simulink model "cntctr"  (R2023b)
settings: Solver=FixedStepDiscrete  StartTime=0.0  StopTime=10.0  FixedStep=0.01  RelTol=1e-3
settings Model: Creator=OWNER  LastModifiedBy=OWNER

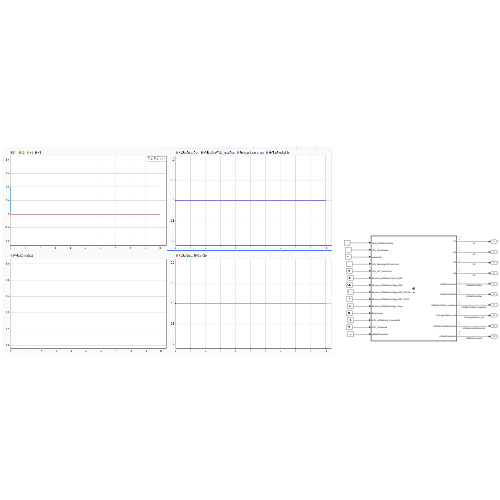
[thumbnail: Simulink's stored preview of the top-level diagram]
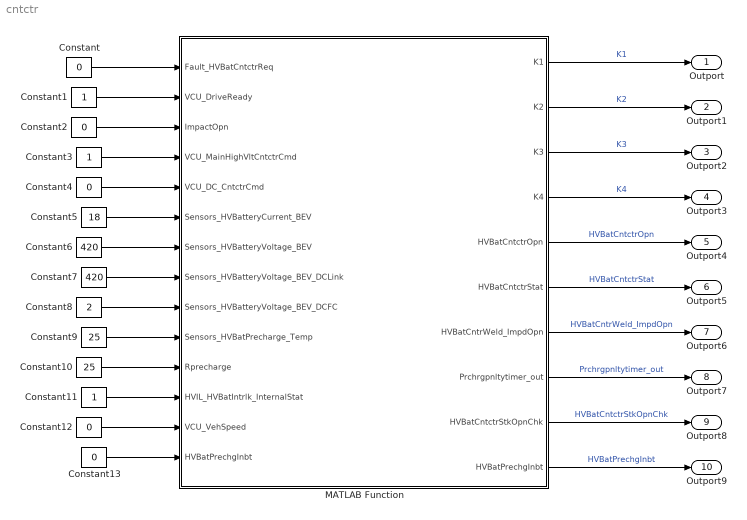
== system cntctr ==
  Constant{,2,4,12..13} (5 alike) : Constant  Value=0
  Constant1 : Constant
  Constant10 : Constant  Value=25
  Constant11 : Constant
  Constant3 : Constant
  Constant5 : Constant  Value=18
  Constant6 : Constant  Value=420
  Constant7 : Constant  Value=420
  Constant8 : Constant  Value=2
  Constant9 : Constant  Value=25
  MATLAB Function : MATLAB Function  TreatAsAtomicUnit=on
  Outport : Outport
  Outport1 : Outport  Port=2
  Outport2 : Outport  Port=3
  Outport3 : Outport  Port=4
  Outport4 : Outport  Port=5
  Outport5 : Outport  Port=6
  Outport6 : Outport  Port=7
  Outport7 : Outport  Port=8
  Outport8 : Outport  Port=9
  Outport9 : Outport  Port=10
  wires:
  Constant/1 -> MATLAB Function/1(Fault_HVBatCntctrReq)
  Constant1/1 -> MATLAB Function/2(VCU_DriveReady)
  Constant2/1 -> MATLAB Function/3(ImpactOpn)
  Constant4/1 -> MATLAB Function/5(VCU_DC_CntctrCmd)
  Constant5/1 -> MATLAB Function/6(Sensors_HVBatteryCurrent_BEV)
  Constant6/1 -> MATLAB Function/7(Sensors_HVBatteryVoltage_BEV)
  Constant7/1 -> MATLAB Function/8(Sensors_HVBatteryVoltage_BEV_DCLink)
  Constant8/1 -> MATLAB Function/9(Sensors_HVBatteryVoltage_BEV_DCFC)
  Constant9/1 -> MATLAB Function/10(Sensors_HVBatPrecharge_Temp)
  Constant10/1 -> MATLAB Function/11(Rprecharge)
  Constant11/1 -> MATLAB Function/12(HVIL_HVBatIntrlk_InternalStat)
  Constant12/1 -> MATLAB Function/13(VCU_VehSpeed)
  Constant13/1 -> MATLAB Function/14("HVBatPrechgInbt ")
  MATLAB Function/1(K1) -> Outport/1  "K1"
  MATLAB Function/2(K2) -> Outport1/1  "K2"
  MATLAB Function/3(K3) -> Outport2/1  "K3"
  MATLAB Function/4(K4) -> Outport3/1  "K4"
  MATLAB Function/5(HVBatCntctrOpn) -> Outport4/1  "HVBatCntctrOpn"
  MATLAB Function/6(HVBatCntctrStat) -> Outport5/1  "HVBatCntctrStat"
  MATLAB Function/7(HVBatCntrWeld_ImpdOpn) -> Outport6/1  "HVBatCntrWeld_ImpdOpn"
  MATLAB Function/8(Prchrgpnltytimer_out) -> Outport7/1  "Prchrgpnltytimer_out"
  MATLAB Function/9(HVBatCntctrStkOpnChk) -> Outport8/1  "HVBatCntctrStkOpnChk"
  MATLAB Function/10(HVBatPrechgInbt) -> Outport9/1  "HVBatPrechgInbt"
  Constant3/1 -> MATLAB Function/4(VCU_MainHighVltCntctrCmd)

== matlab function cntctr/MATLAB Function ==
  data: Fault_HVBatCntctrReq input; K1 output; VCU_DriveReady input; ImpactOpn input; VCU_MainHighVltCntctrCmd input; VCU_DC_CntctrCmd input; Sensors_HVBatteryCurrent_BEV input; Sensors_HVBatteryVoltage_BEV input; Sensors_HVBatteryVoltage_BEV_DCLink input; Sensors_HVBatteryVoltage_BEV_DCFC input; Sensors_HVBatPrecharge_Temp input; Rprecharge input; HVIL_HVBatIntrlk_InternalStat input; VCU_VehSpeed input; HVBatPrechgInbt input; K2 output; K3 output; K4 output; HVBatCntctrOpn output; HVBatCntctrStat output; HVBatCntrWeld_ImpdOpn output; Prchrgpnltytimer_out output; HVBatCntctrStkOpnChk output; HVBatPrechgInbt output
function [K1, K2, K3, K4, HVBatCntctrOpn, HVBatCntctrStat, HVBatCntrWeld_ImpdOpn, Prchrgpnltytimer_out, HVBatCntctrStkOpnChk, HVBatPrechgInbt] = fcn(Fault_HVBatCntctrReq, VCU_DriveReady, ImpactOpn, VCU_MainHighVltCntctrCmd, VCU_DC_CntctrCmd, Sensors_HVBatteryCurrent_BEV, Sensors_HVBatteryVoltage_BEV, Sensors_HVBatteryVoltage_BEV_DCLink, Sensors_HVBatteryVoltage_BEV_DCFC, Sensors_HVBatPrecharge_Temp, Rprecharge, HVIL_HVBatIntrlk_InternalStat, VCU_VehSpeed, HVBatPrechgInbt)
%-----------------------------------------------------------
% McMaster Automotive Resource Centre (MARC)
% Electrical Engineer: Romulo Vieira, M.Sc and MBA - PhD Candidate
%-----------------------------------------------------------
% Purpose: Manage precharge relay and contactor sequence with retry + inhibit logic
%-----------------------------------------------------------
% HVBatCntctrStat Mapping:
% 0 – Idle/Waiting
% 1 – Precharge Active
% 2 – Precharge Complete (Main contactors closed)
% 3 – Precharge Failed (necessary cooldown after unique failures of voltage and current)
% 4 – Inhibit State (necessary cooldown after multiple failures)
% 5 - DCFC Charging
% 6 – Contactor Control Shorted High
% 7 - Contactor Control Shorted Low
% VCU_MainHighVltCntctrCmd mapping:
% 0 - open
% 1 - closed
% 2 - impact_open
% 3 - fast_open
% 7 - invalid
% HVBatCntrWeld_ImpdOpn (Contactor welded and has impeded opening when commanded by BPCM) Mapping:
% 0: Normal
% 1: Stuck_Open
% 2: Stuck_Closed
% 3: SNA
% --- Constants ---
Unset_VbusTargetHitIdx             = -1;   % Flag indicating Vbus threshold not yet hit
Min_Samples                        = 0;    % Minimum number of samples where relays and contactor are both active
% Internal Configuration Parameters
Ke_t_PrechargeFailCoolTime             = 1000;   % Cooldown time after one single failed attempt [ms]
Ke_t_ExtraPrechargeFailCoolPenaltyTime = 1000;   % Additional cooldown after two multiple failures [ms]
Ke_t_PrechargeFailMaxPenalty           = 10000;  % Maximum time threshold before enabling precharge inhibit state
Ke_t_BPCM_Precharge_Fail_Penalty_Time  = 15000;  % Hard inhibit time if failures persist [ms]
Ke_I_HighVoltageBusShortageCurrentMin  = 10.8;   % Minimum expected precharge current [A] (Pack current ≥ 0.6 * (pack voltage / Precharge resistance))
                                                 % // max pack voltage = 450 V, Precharge resistance = 25 ohm
Ke_V_HighVoltagePreChargeThreshold     = 0.98 * Sensors_HVBatteryVoltage_BEV;  % Target voltage threshold
Ke_t_HighVoltageBusPrechargeTime       = 300;    % Maximum allowable time for precharging [ms]
Ke_b_WeldCheckEnabler                  = 1;      % Check if weld check diagnostic is enabled (0 - disabled, 1 - enabled)
Ke_v_WeldCheckEnableSpeed              = 5;      % km/h 


%% Add a delay for shorted high/stuck closed
stuck_closed_delay = 10000; % 10000 milliseconds

% --- Persistent Variables ---
persistent I_buffer idx HVBatCntctrStat_Aux VbusTargetHitIdx ...
    t_counter last_PrechargeAllw Prchrgpnltytimer PrechargeFailCount last_HVBatCntctrStat_Aux HVBatCntrWeld_ImpdOpn_Aux Ke_b_WeldCheckEnabler_Aux stuck_closed_delay_Timer
if isempty(I_buffer)
    I_buffer               = zeros(Ke_t_HighVoltageBusPrechargeTime,1);
    idx                    = 1;
    HVBatCntctrStat_Aux    = 0;
    VbusTargetHitIdx       = Unset_VbusTargetHitIdx;
    t_counter              = 0;
    last_PrechargeAllw     = 0;
    Prchrgpnltytimer       = 0;
    PrechargeFailCount     = 0; % Represented by k_fail in the flowchart
    last_HVBatCntctrStat_Aux = 0;
    HVBatCntrWeld_ImpdOpn_Aux = 0;
    Ke_b_WeldCheckEnabler_Aux = 1;
    stuck_closed_delay_Timer = 15000;
end
% --- Default Outputs ---
K1 = 0; K2 = 0; K3 = 0; K4 = 0;
HVBatCntctrStat = HVBatCntctrStat_Aux;
Ke_t_HighVoltageBusActualPrechargeTime = 0;
Ke_I_HighVoltageBusShortageCurrent = 0;
HVBatCntctrStkOpnChk = 0;
%-----------------------------------------------------------
% Weld Check Enable Logic (Explicit & Robust)
%
% Weld check is ENABLED only when:
% - Contactor command is NOT IMPACT_OPEN
% - AND (Contactor command is NOT OPEN
%        OR Vehicle speed <= threshold)
%-----------------------------------------------------------

if VCU_MainHighVltCntctrCmd == 2 || ImpactOpn == 1
    % IMPACT_OPEN → permanently disable weld check
    Ke_b_WeldCheckEnabler_Aux = 0;

elseif (VCU_MainHighVltCntctrCmd == 0) && ...
       (VCU_VehSpeed > Ke_v_WeldCheckEnableSpeed)
    % OPEN + vehicle moving → temporarily disable
    Ke_b_WeldCheckEnabler_Aux = 0;

else
    % All other conditions → weld check allowed
    Ke_b_WeldCheckEnabler_Aux = 1;
    HVBatCntctrStkOpnChk = 1;
end

% FAST_OPEN handling (state reset only)
if VCU_MainHighVltCntctrCmd == 3 || ImpactOpn == 1
    HVBatCntctrStat_Aux = 0;
end

% IMPACT_OPEN must also force state reset
if VCU_MainHighVltCntctrCmd == 2 || ImpactOpn == 1
    HVBatCntctrStat_Aux = 0;
end


% --- State Machine ---
switch HVBatCntctrStat_Aux
    case 0 % OPEN STATE
        HVBatCntctrOpn = 0;
        % Set the Battery Contactor States
        K1 = 0; K2 = 0; K3 = 0; K4 = 0;
        % Check Initial conditions
        % HVIL_HVBatIntrlk_InternalStat = 1 (pass),
        % HVIL_HVBatIntrlk_InternalStat = 2 (fail)
        % For precharge initiation HVIL_HVBatIntrlk_InternalStat must pass.
        if VCU_MainHighVltCntctrCmd == 1 && HVBatPrechgInbt == 0 && HVIL_HVBatIntrlk_InternalStat == 1 && Fault_HVBatCntctrReq == 0 && Sensors_HVBatPrecharge_Temp < 60
            I_buffer(:) = 0;
            idx = 1;
            VbusTargetHitIdx = Unset_VbusTargetHitIdx;
            t_counter = 0;
            HVBatCntctrStat_Aux = 1;
        end

        %% Shorted High
        
        if VCU_MainHighVltCntctrCmd == 0 && Sensors_HVBatteryVoltage_BEV_DCLink > 270 && Ke_b_WeldCheckEnabler_Aux == 1 
            stuck_closed_delay_Timer = stuck_closed_delay_Timer - 1;
            if stuck_closed_delay_Timer == 0
                HVBatCntctrStat_Aux = 6;
                HVBatCntrWeld_ImpdOpn_Aux = 2; 
            end
        end

    case 1  % PRECHARGING STATE
        HVBatCntctrOpn = 0;
        % Abort if initial conditions are no longer valid
        if VCU_MainHighVltCntctrCmd == 0 || HVBatPrechgInbt == 1 || HVIL_HVBatIntrlk_InternalStat == 2 || Fault_HVBatCntctrReq == 1 || Sensors_HVBatPrecharge_Temp >= 60
            HVBatCntctrStat_Aux = 0;
        end
        % Set precharge relays ON
        K1 = 0; K2 = 1; K3 = 1; K4 = 0;
        %
        % if Fault_K1_Shorted_Low_Condition == 1
        %     HVBatCntctrStat_Aux = 7; % K1 Shorted Low
        % end
        % if Fault_K4_Shorted_Low_Condition == 1
        %     HVBatCntctrStat_Aux = 7; % K4 Shorted Low
        % end
        % Record current
        if t_counter == 0
            I_buffer(idx) = Sensors_HVBatteryVoltage_BEV / Rprecharge;
        else
            I_buffer(idx) = Sensors_HVBatteryCurrent_BEV;
        end
        Ke_I_HighVoltageBusShortageCurrent = max(I_buffer);
        % Voltage target check
        if VbusTargetHitIdx == Unset_VbusTargetHitIdx && Sensors_HVBatteryVoltage_BEV_DCLink >= Ke_V_HighVoltagePreChargeThreshold
            VbusTargetHitIdx = t_counter + 1;
        end
        % Time since start or since target hit
        if VbusTargetHitIdx ~= Unset_VbusTargetHitIdx
            delta_samples = VbusTargetHitIdx;
        else
            delta_samples = t_counter;
        end
        % SUCCESS - PRECHARGE CONDITIONS ARE MET
        if t_counter < Ke_t_HighVoltageBusPrechargeTime && ...
                VbusTargetHitIdx ~= Unset_VbusTargetHitIdx && delta_samples < Ke_t_HighVoltageBusPrechargeTime && Ke_I_HighVoltageBusShortageCurrent >= Ke_I_HighVoltageBusShortageCurrentMin
            
            % Set the next Battery Contactor Status
            HVBatCntctrStat_Aux = 2;
            % Set the Battery Contactor States
            K1 = 1; K2 = 0; K3 = 0; K4 = 0;
            PrechargeFailCount = 0;
            Prchrgpnltytimer = 0;
        % FAILURE - PRECHARGE CONDITIONS ARE NOT MET
        elseif t_counter == Ke_t_HighVoltageBusPrechargeTime && ...
               (VbusTargetHitIdx == Unset_VbusTargetHitIdx || delta_samples == Ke_t_HighVoltageBusPrechargeTime || Ke_I_HighVoltageBusShortageCurrent < Ke_I_HighVoltageBusShortageCurrentMin)
            % Set the Battery Contactor States
            K1 = 0; K2 = 0; K3 = 0; K4 = 0;
           % Set the Battery Contactor Status
            HVBatCntctrStat_Aux = 3;
            % Update the total cooling time before re-attempt
            PrechargeFailCount = PrechargeFailCount + 1;
            Prchrgpnltytimer = Prchrgpnltytimer + Ke_t_PrechargeFailCoolTime;
            if PrechargeFailCount >= 2
                Prchrgpnltytimer = Ke_t_ExtraPrechargeFailCoolPenaltyTime;
            end
            if PrechargeFailCount >= 10
                HVBatCntctrStat_Aux = 4;
                HVBatPrechgInbt = 1;
                Prchrgpnltytimer = Ke_t_BPCM_Precharge_Fail_Penalty_Time;
            end
        end
        % Update counters
        t_counter = t_counter + 1;
        idx = idx + 1;
        if idx > Ke_t_HighVoltageBusPrechargeTime, idx = 1; end
    case 2  % PRECHARGE COMPLETE OR CLOSED
        HVBatCntctrOpn = 0;
        % Set the Battery Contactor States
        K1 = 1; K2 = 0; K3 = 0; K4 = 0;
        % If statement to detect DCFC charging
        if VCU_DC_CntctrCmd == 1
            HVBatCntctrStat_Aux = 5; % DCFC CHARGING
        end
        if VCU_MainHighVltCntctrCmd == 0
            HVBatCntctrStat_Aux = 0;
        end

        if VCU_MainHighVltCntctrCmd == 1 && Sensors_HVBatteryVoltage_BEV_DCLink < 270 && Ke_b_WeldCheckEnabler_Aux == 1
            HVBatCntctrStat_Aux = 7;
            HVBatCntrWeld_ImpdOpn_Aux = 1;
        end

    case 3 % FAULT: PRECHARGE FAILED STATE 4 --> 3
        HVBatCntctrOpn = 1;
        % Set the Battery Contactor States
        K1 = 0; K2 = 0; K3 = 0; K4 = 0;
        if Prchrgpnltytimer > 0
            Prchrgpnltytimer = Prchrgpnltytimer - 1;
        else
            HVBatCntctrStat_Aux = 0;
        end
    case 4  % FAULT: PRECHARGE INHIBIT STATE - 5 -- > 4
        HVBatCntctrOpn = 1;
        % Set the Battery Contactor States
        K1 = 0; K2 = 0; K3 = 0; K4 = 0;
        if Prchrgpnltytimer > 0
            Prchrgpnltytimer = Prchrgpnltytimer - 1;
        else
            Prchrgpnltytimer = 0;
            HVBatPrechgInbt = 0;
            HVBatCntctrStat_Aux = 0;
            PrechargeFailCount = 0;
        end
    case 5 % DCFC CHARGING
        HVBatCntctrOpn = 0;
        % Set the Battery Contactor States
        K1 = 1; K2 = 0; K3 = 0; K4 = 1;
        if VCU_DC_CntctrCmd == 0
            if VCU_MainHighVltCntctrCmd == 0
                HVBatCntctrStat_Aux = 0; % switch to OPEN
            else
                HVBatCntctrStat_Aux = 2; % switch to CLOSED
            end
        end
    
    case 6 % FAULT: Shorted High
        HVBatCntctrOpn = 1;
        if VCU_MainHighVltCntctrCmd == 0 && Sensors_HVBatteryVoltage_BEV_DCLink < 270
            HVBatCntctrStat_Aux = 0;
            HVBatCntrWeld_ImpdOpn_Aux = 0;
        end

    case 7 % FAULT: Shorted Low
        HVBatCntctrOpn = 1;
        if VCU_DC_CntctrCmd == 0 && Sensors_HVBatteryVoltage_BEV_DCFC < 270 && VCU_MainHighVltCntctrCmd == 1 && Sensors_HVBatteryVoltage_BEV_DCLink > 270
            HVBatCntctrStat_Aux = 2;
            HVBatCntrWeld_ImpdOpn_Aux = 0;
        end
    otherwise
        HVBatCntctrOpn = 1;
        K1 = 0; K2 = 0; K3 = 0; K4 = 0;
        HVBatCntctrStat_Aux = 0;
end
% --- Final Outputs ---
HVBatCntctrStat = HVBatCntctrStat_Aux;
HVBatCntrWeld_ImpdOpn = HVBatCntrWeld_ImpdOpn_Aux;
Ke_b_WeldCheckEnabler = Ke_b_WeldCheckEnabler_Aux;
Ke_t_HighVoltageBusActualPrechargeTime = max(0, VbusTargetHitIdx + ...
    Min_Samples * (VbusTargetHitIdx ~= Unset_VbusTargetHitIdx));
Prchrgpnltytimer_out = Prchrgpnltytimer;
last_PrechargeAllw = double(Fault_HVBatCntctrReq);
last_HVBatCntctrStat_Aux = HVBatCntctrStat_Aux;
end
